simulink model "GRPsimNoDragModel"  (R2024b)
settings: Solver=VariableStepAuto  StartTime=0.0  StopTime=30  RelTol=1e-3
libraries: shared6dof x1, simulink x1
settings Model: Creator=aniketray  LastModifiedBy=aniketray

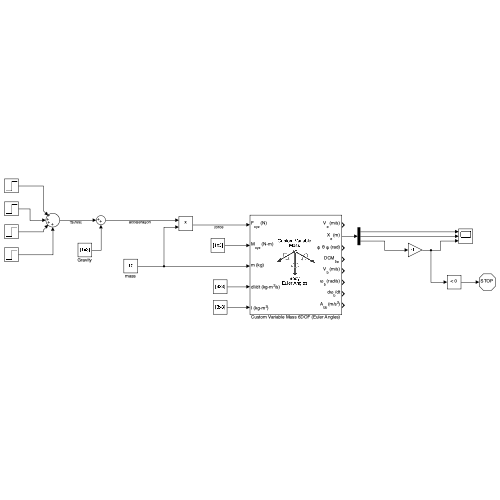
[thumbnail: Simulink's stored preview of the top-level diagram]
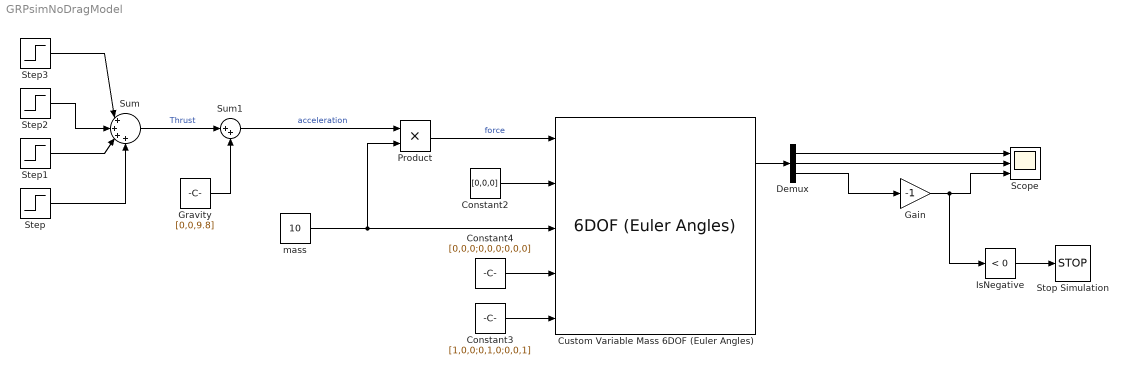
== system GRPsimNoDragModel ==
  Constant2 : Constant  Value=[0,0,0]
  Constant3 : Constant  Value=[1,0,0;0,1,0;0,0,1]
  Constant4 : Constant  Value=[0,0,0;0,0,0;0,0,0]
  Custom Variable Mass 6DOF (Euler Angles) : shared6dof/6DOF (Euler Angles)  units=Metric (MKS)  mtype=Custom Variable  rep=Euler Angles  xme_0=[0 0 0]  Vm_0=[0 0 0]  eul_0=[0 0 0]  pm_0=[0 0 0]  mass_0=1.0  mass_e=0.5  mass_f=2.0  inertia=eye(3)  inertia_e=eye(3)  inertia_f=2*eye(3)  k_quat=1.0  vre_flag=off  abi_flag=off  aMode=0  xme_statename=''  Vm_statename=''  eul_statename=''  quat_statename=''  pm_statename=''  mass_statename=''
      settings: LibrarySourceBlock=aerolib6dof2/Custom Variable Mass 6DOF (Euler Angles)
  Demux : Demux  Outputs=3
  Gain : Gain  Gain=-1
  Gravity : Constant  Value=[0,0,9.8]
  IsNegative : simulink/Logic and Bit Operations/Compare To Zero  relop=<  OutDataTypeStr=boolean
      settings: LibrarySourceBlock=|
      | simulink/Quick Insert/Logic and Bit
      | Operations/IsNegative
  Product : Product
  Scope : Scope  NumInputPorts=3
  Step : Step  Time=0  After=[0,0,-15]  SampleTime=0.001
  Step1 : Step  Time=3  After=[0,0,15]  SampleTime=0.001
  Step2 : Step  Time=6.18367346939  After=[0,0,-15]  SampleTime=0.001
  Step3 : Step  Time=9.18367346939  After=[0,0,15]  SampleTime=0.001
  Stop Simulation : Stop
  Sum : Sum  Inputs=|++++
  Sum1 : Sum  Inputs=|++
  mass : Constant  Value=10
  wires:
  mass/1 -> Product/2, Custom Variable Mass 6DOF (Euler Angles)/3
  Constant2/1 -> Custom Variable Mass 6DOF (Euler Angles)/2
  Constant3/1 -> Custom Variable Mass 6DOF (Euler Angles)/5
  Constant4/1 -> Custom Variable Mass 6DOF (Euler Angles)/4
  Product/1 -> Custom Variable Mass 6DOF (Euler Angles)/1  "force"
  Custom Variable Mass 6DOF (Euler Angles)/2 -> Demux/1
  Demux/1 -> Scope/1
  Demux/2 -> Scope/2
  Demux/3 -> Gain/1
  Gain/1 -> IsNegative/1, Scope/3
  IsNegative/1 -> Stop Simulation/1
  Step/1 -> Sum/4
  Step1/1 -> Sum/3
  Step2/1 -> Sum/2
  Step3/1 -> Sum/1
  Sum/1 -> Sum1/1  "Thrust"
  Gravity/1 -> Sum1/2
  Sum1/1 -> Product/1  "acceleration"
